simulink model "PCMPWMDEMO"  (R2014b)
settings: Solver=FixedStepDiscrete  StartTime=0.0  StopTime=10.0  FixedStep=8e-4  RelTol=1e-3
PreLoadFcn:
  | Hyo_customization
libraries: periblklib x3
settings Model: Creator=Hyowinner  LastModifiedBy=sunzx.fnst
settings OptimizationCC: InlineParams=on  OptimizeModelRefInitCode=on  LifeSpan=1
settings HardwareCC: ProdLargestAtomicInteger=Integer  ProdLargestAtomicFloat=Float  ProdIntDivRoundTo=Zero  ProdEndianess=LittleEndian  ProdHWDeviceType=CYPRESS->ARM Cortex-R5
settings RTWCC: SystemTargetFile=Hyo.tlc  GenCodeOnly=on  MakeCommand=none  GenerateMakefile=off  TemplateMakefile=none  Description=System Target File for S6J3200 Series MCU Target  GenerateReport=on  ProcessScript=Hyo_make_rtw_hook  IncludeHyperlinkInReport=on  LaunchReport=on
settings CodeAppCC: IgnoreCustomStorageClasses=off
settings STFCustomTargetCC: ModelReferenceCompliant=off  IncludeMdlTerminateFcn=off  CombineOutputUpdateFcns=on  ERTFirstTimeCompliant=on  ERTCustomFileBanners=on  SupportContinuousTime=off  SupportNonInlinedSFcns=off  MATLABClassNameForMDSCustomization=Simulink.SoftwareTarget.ERTCustomization  GRTInterface=off  SystemTargetFile=Hyo.tlc
settings ERTTargetCC: ModelReferenceCompliant=off  ParMdlRefBuildCompliant=off  CompOptLevelCompliant=off  ConcurrentExecutionCompliant=off  IncludeMdlTerminateFcn=off  ModelStepFunctionPrototypeControlCompliant=off  CPPClassGenCompliant=off  InlinedParameterPlacement=NonHierarchical  ERTSrcFileBannerTemplate=Hyo_code_template.cgt  ERTHdrFileBannerTemplate=Hyo_code_template.cgt  ERTDataSrcFileTemplate=Hyo_code_template.cgt  ERTDataHdrFileTemplate=Hyo_code_template.cgt  ERTCustomFileTemplate=Hyo_file_process.tlc  EnableUserReplacementTypes=on

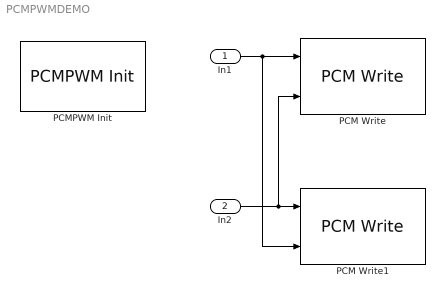
== system PCMPWMDEMO ==
  In1 : Inport
  In2 : Inport  Port=2
  PCM Write : periblklib/PCMPWM/PCM Write  g_pv=s6j3200_PCMPWM.h,PCMPWM,_Write_5;datregnum,5;stereomode,stereo mode;
  PCM Write1 : periblklib/PCMPWM/PCM Write  g_pv=s6j3200_PCMPWM.h,PCMPWM,_Write_12;datregnum,12;stereomode,stereo mode;
  PCMPWM Init : periblklib/PCMPWM/PCMPWM Init  g_pv=s6j3200_PCMPWM.h,PCMPWM,_Init;deadtimeval,0;fifoempnum,45;doublemode,off;opmpd,low-pass filter;stereomode,stereo mode;debugmode,off;dmamode,off;silencemode,off;outlvlselch1,PCMPWM_1_AH/BH are high-active and PCMPWM_1_AL/BL are low-active;outlvlselch0,PCMPWM_0_AH/BH are high-active and PCMPWM_0_AL/BL are low-active;outputench1,PCMPWM_1_AH/BH/AL/BL are set to the inactive value;outputench0,PCMPWM_0_AH/BH/AL/BL are set to the inactive value;clksel,Divide by 4: Conversion counter clock = PWM_CLK/4;cntperiod,35;pcmoffset,257;dmablkerrorint,off;fifoundrunerr,off;fifoovflerr,off;datareqerr,off;enpcmpwm,on;an0al0,P4_30;an1al1,P5_02;ap0ah0,P4_29;ap1ah1,P5_01;bn0bl0,P5_00;bn1bl1,P5_04;bp0bh0,P4_31;bp1bh1,P3_27;
  wires:
  In1/1 -> PCM Write1/2, PCM Write/1
  In2/1 -> PCM Write/2, PCM Write1/1
